simulink model "Unwucht4_Frequenzgang"  (R2018b)
settings: Solver=VariableStepAuto  StartTime=0.0  StopTime=40  RelTol=1e-3
values from neighbouring files (symbols this model uses):
  a1T = a1T{:}    [Unwuchterregung_Anlauf.m]    (also in Unwuchterregung_mit_Tilger.m)
  a2T = a2T{:}    [Unwuchterregung_Anlauf.m]    (also in Unwuchterregung_mit_Tilger.m)
  b1T = b1T{:}    [Unwuchterregung_Anlauf.m]    (also in Unwuchterregung_mit_Tilger.m)
  b2T = b2T{:}    [Unwuchterregung_Anlauf.m]    (also in Unwuchterregung_mit_Tilger.m)
  mu = 24+wasser    (= 49)    [Unwuchterregung_Anlauf.m]    (also in Unwuchterregung_mit_Tilger.m; Unwuchterregung_ohne_ST.m)
  ru = 0.330    (= 0.33)    [Unwuchterregung_Anlauf.m]    (also in Unwuchterregung_mit_Tilger.m; Unwuchterregung_ohne_ST.m)
settings Model: Creator=avsto  LastModifiedBy=avsto

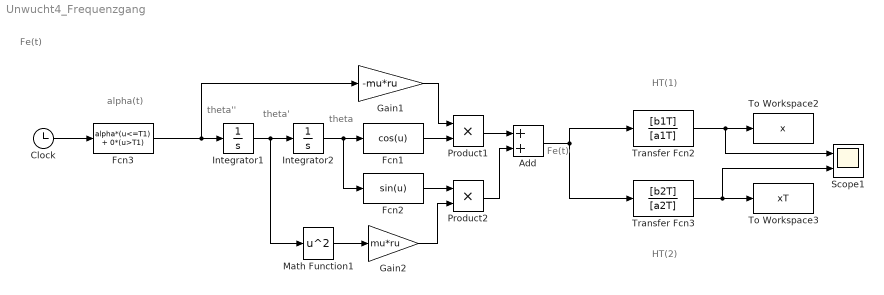
== system Unwucht4_Frequenzgang ==
  note: theta''
  note: Fe(t)
  note: theta
  note: HT(1)
  note: alpha(t)
  note: Fe(t)
  note: HT(2)
  note: theta'
  Add : Sum
  Clock : Clock
      settings: Decimation=1000
  Fcn1 : Fcn  Expr=cos(u)
  Fcn2 : Fcn  Expr=sin(u)
  Fcn3 : Fcn  Expr=alpha*(u<=T1) + 0*(u>T1)
  Gain1 : Gain  Gain=-mu*ru
  Gain2 : Gain  Gain=mu*ru
  Integrator1 : Integrator
  Integrator2 : Integrator
  Math Function1 : Math  Operator=square  SaturateOnIntegerOverflow=on
  Product1 : Product  RndMeth=Zero
  Product2 : Product  RndMeth=Zero
  Scope1 : Scope  NumInputPorts=2
  To Workspace2 : ToWorkspace  VariableName=x  SaveFormat=Structure With Time  SampleTime=-1
  To Workspace3 : ToWorkspace  VariableName=xT  SaveFormat=Structure With Time  SampleTime=-1
  Transfer Fcn2 : TransferFcn  Numerator=[b1T]  Denominator=[a1T]
  Transfer Fcn3 : TransferFcn  Numerator=[b2T]  Denominator=[a2T]
  wires:
  Transfer Fcn3/1 -> Scope1/2, To Workspace3/1
  Transfer Fcn2/1 -> Scope1/1, To Workspace2/1
  Math Function1/1 -> Gain2/1
  Product2/1 -> Add/2
  Clock/1 -> Fcn3/1
  Gain2/1 -> Product2/2
  Fcn3/1 -> Gain1/1, Integrator1/1
  Product1/1 -> Add/1
  Integrator2/1 -> Fcn2/1, Fcn1/1
  Integrator1/1 -> Math Function1/1, Integrator2/1
  Gain1/1 -> Product1/1
  Add/1 -> Transfer Fcn3/1, Transfer Fcn2/1
  Fcn2/1 -> Product2/1
  Fcn1/1 -> Product1/2
